simulink model "IonSatSimulationD"  (R2020b)
settings: Solver=ode3  StartTime=0.0  StopTime=t_sim  FixedStep=TimeStep  MaxStep=30  MinStep=.1  RelTol=1e-3
model workspace (MAT data in the model file):
  repartition_matrix : Simulink.Parameter (value not decoded)
  wheel_number : Simulink.Parameter (value not decoded)
values from neighbouring files (symbols this model uses):
  MODE = 4    [Full_model_PID_MEKF_Scenario1_Monte_Carlo.m]    (also in Full_model_PID_MEKF_Scenario3_Monte_Carlo.m = MODE_SEQUENCE(1); Full_model_PID_UKF_Scenario1_Monte_Carlo.m; Full_model_PID_UKF_Scenario2_Monte_Carlo.m = 2; Full_model_PID_UKF_Scenario3_Monte_Carlo.m = MODE_SEQUENCE(1))
  Use_IGRF = 1    [Full_model_PID_MEKF_Scenario1_Monte_Carlo.m]    (also in Full_model_PID_MEKF_Scenario3_Monte_Carlo.m; Full_model_PID_UKF_Scenario1_Monte_Carlo.m; Full_model_PID_UKF_Scenario2_Monte_Carlo.m; Full_model_PID_UKF_Scenario3_Monte_Carlo.m)
  Use_IGRF_KF = 1    [Full_model_PID_MEKF_Scenario1_Monte_Carlo.m]    (also in Full_model_PID_MEKF_Scenario3_Monte_Carlo.m; Full_model_PID_UKF_Scenario1_Monte_Carlo.m; Full_model_PID_UKF_Scenario2_Monte_Carlo.m; Full_model_PID_UKF_Scenario3_Monte_Carlo.m)
undefined symbols (not defined in the file or in its folder): att, date, deg, DiscIntNeverNeededParam, IonSataero, km, m, orbit, rad, s, sat
libraries: aerolibutil x30, vrlib x19, aerolibconvert2 x13, dspmathops x13, sharedtransform x12, simulink x10, sharedutil x5, DipoleModel x3, aerolibobsolete x3, simulink_extras x2, aerolibcelestial x2, dspstat3 x1
(part 3 of 3)

== system IonSatSimulationD/Sensors/Sun Sensor (Sun sensor) ==
  note: Two sensors because the top-camera has a 3-sigma=0.2° wheread the coarse sun sensors have sigma = 10°
  note: Valeur constructeur : 3-sigma = 0.2°
      | Donc sigma = 0.066° = 0.001164 rad
  note: Test d'eclipse
  note: Tests if the camera is seeing the sun
  Sat-Sun_ECI : Inport
  U : Inport  Port=2
  AND1 : Logic  IconShape=distinctive  AllPortsSameDT=off  OutDataTypeStr=boolean
  Bus Selector : BusSelector  OutputSignals=Q_ECI,XYZ_ECI
  Constant3 : Constant  Value=true
  Constant4 : Constant  Value=false
  Demux : Demux  Outputs=3
  Eclipse Test 0: in eclipse 1: illumination : MATLABFcn  MATLABFcn=eclipse_check
  Manual Switch : ManualSwitch
  Mux : Mux  Inputs=2
  Quaternion Rotation : aerolibutil/Quaternion Rotation
  Quaternion Rotation1 : aerolibutil/Quaternion Rotation
  Random Number : RandomNumber  Mean=[0 0 0]  Variance=sat.sensors.sun_sigma*sat.sensors.sun_sigma  Seed=[0 5 355]  SampleTime=1  VectorParams1D=off
  Rotation Angles to Quaternions : sharedtransform/Rotation Angles to Quaternions  rotationOrder=ZYX  aMode=aMode
      settings: SourceProductBaseCode=AE,PW,MT,UV,VE,VP
  Switch : Switch  Criteria=u2 > Threshold
  Terminator : Terminator
  Terminator1 : Terminator
  switch here to never have an eclipse : Constant
  Sat-Sun_precise_body_meas : Outport  VectorParamsAs1DForOutWhenUnconnected=off
  Sensor active (bool) : Outport  Port=2  VectorParamsAs1DForOutWhenUnconnected=off
  wires:
  Rotation Angles to Quaternions/1 -> Quaternion Rotation/1
  Quaternion Rotation/1 -> Sat-Sun_precise_body_meas/1
  U/1 -> Bus Selector/1
  Bus Selector/1 -> Quaternion Rotation1/1  "<Q_ECI>"
  Quaternion Rotation1/1 -> Demux/1, Quaternion Rotation/2  "Sat_Sun_body"
  Demux/3 -> Switch/2
  Constant3/1 -> Switch/1
  Demux/2 -> Terminator/1
  Demux/1 -> Terminator1/1
  Random Number/1 -> Rotation Angles to Quaternions/1
  Constant4/1 -> Switch/3
  Mux/1 -> Eclipse Test 0: in eclipse 1: illumination/1
  AND1/1 -> Manual Switch/1
  Bus Selector/2 -> Mux/1  "<XYZ_ECI>"
  Eclipse Test 0: in eclipse 1: illumination/1 -> AND1/2
  Switch/1 -> AND1/1
  Sat-Sun_ECI/1 -> Mux/2, Quaternion Rotation1/2
  switch here to never have an eclipse/1 -> Manual Switch/2
  Manual Switch/1 -> Sensor active (bool)/1

== system IonSatSimulationD/Attitude Controller/B-dot choice1/Switch Case Action Subsystem3 ==
  In1 : Inport
  Action Port : ActionPort  ActionPortLabel=if(u1 > 0)
  Out1 : Outport  VectorParamsAs1DForOutWhenUnconnected=off
  wires:
  In1/1 -> Out1/1

== system IonSatSimulationD/Attitude Controller/B-dot choice1/Switch Case Action Subsystem4 ==
  In1 : Inport
  Action Port : ActionPort  ActionPortLabel=else
  Out1 : Outport  VectorParamsAs1DForOutWhenUnconnected=off
  wires:
  In1/1 -> Out1/1

== system IonSatSimulationD/Attitude Controller/B-dot choice2/Switch Case Action Subsystem3 ==
  In1 : Inport
  Action Port : ActionPort  ActionPortLabel=if(u1 > 0)
  Out1 : Outport  VectorParamsAs1DForOutWhenUnconnected=off
  wires:
  In1/1 -> Out1/1

== system IonSatSimulationD/Attitude Controller/B-dot choice2/Switch Case Action Subsystem4 ==
  In1 : Inport
  Action Port : ActionPort  ActionPortLabel=else
  Out1 : Outport  VectorParamsAs1DForOutWhenUnconnected=off
  wires:
  In1/1 -> Out1/1

== system IonSatSimulationD/Attitude Controller/PID (nominal command)/Command Magnetic moments computation ==
  note: Moment magnétique de commande M :
      |
      | $M_c = \frac{1}{B²}\vec{B} \wedge\vec{T_P}$
      |
      | Avec Tp couple projeté dans le plan orthogonal à B
      | $T_P=\vec{T}-\frac{1}{B²}(\vec{T}\cdot\vec{B})\vec{B}$
  Command (vect) : Inport  OutDataTypeStr=double
  B_IGRF_body (vect) : Inport  Port=2  OutDataTypeStr=double
  h1 (vect) : Inport  Port=3
  h2 (vect) : Inport  Port=4
  h3 (vect) : Inport  Port=5
  Cross Product : vrlib/Utilities/Cross Product
  Dot Product : DotProduct  InputSameDT=on  OutDataTypeStr=Inherit: Inherit via internal rule
  Global magnetic moment computation : Subsystem
  Mux : Mux  Inputs=3
  Product1 : Product  Inputs=*/
  Reshape : Reshape  OutputDimensionality=Column vector (2-D)
  Reshape1 : Reshape  OutputDimensionality=Column vector (2-D)
  Mag vector command : Outport  VectorParamsAs1DForOutWhenUnconnected=off
  wires:
  B_IGRF_body (vect)/1 -> Reshape1/1  "B_Body"
  Command (vect)/1 -> Reshape/1  "T_Body"
  h1 (vect)/1 -> Global magnetic moment computation/2(In2)
  h2 (vect)/1 -> Global magnetic moment computation/3(In3)
  h3 (vect)/1 -> Global magnetic moment computation/4(In4)
  Global magnetic moment computation/2(magnetic moment 2 (scalar)) -> Mux/2  "magnetic moment 2"
  Global magnetic moment computation/3(magnetic moment 3 (scalar)) -> Mux/3  "magnetic moment 3"
  Global magnetic moment computation/1(magnetic moment 1 (scalar)) -> Mux/1  "magnetic moment 1"
  Mux/1 -> Mag vector command/1
  Reshape1/1 -> Cross Product/2, Dot Product/2, Dot Product/1
  Cross Product/1 -> Product1/1
  Product1/1 -> Global magnetic moment computation/1(In1)  "Mc"
  Dot Product/1 -> Product1/2  "B^2"
  Reshape/1 -> Cross Product/1  "Tp"

== system IonSatSimulationD/Attitude Controller/PID (nominal command)/Extract Vect ==
  Qr : Inport
  Demux : Demux
  Mux1 : Mux  Inputs=3
  Product : Product
  Reshape : Reshape  OutputDimensionality=Column vector (2-D)
  Sign : Signum
  Qvect : Outport  VectorParamsAs1DForOutWhenUnconnected=off
  wires:
  Demux/2 -> Mux1/1
  Demux/4 -> Mux1/3
  Demux/3 -> Mux1/2
  Demux/1 -> Sign/1
  Qr/1 -> Demux/1
  Mux1/1 -> Product/2
  Product/1 -> Reshape/1
  Sign/1 -> Product/1
  Reshape/1 -> Qvect/1

== system IonSatSimulationD/Attitude Controller/PID (nominal command)/If Action Subsystem ==
  In1 : Inport
  Action Port : ActionPort  ActionPortLabel=else
  Out1 : Outport  VectorParamsAs1DForOutWhenUnconnected=off
  wires:
  In1/1 -> Out1/1

== system IonSatSimulationD/Attitude Controller/PID (nominal command)/If Action Subsystem1 ==
  In1 : Inport
  Action Port : ActionPort  ActionPortLabel=if(u1 > 0)
  Out1 : Outport  VectorParamsAs1DForOutWhenUnconnected=off
  wires:
  In1/1 -> Out1/1

== system IonSatSimulationD/Attitude Controller/PID (nominal command)/If Action Subsystem2 ==
  In1 : Inport
  Action Port : ActionPort  ActionPortLabel=if(u1 > 0.0068)
  Out1 : Outport  VectorParamsAs1DForOutWhenUnconnected=off
  wires:
  In1/1 -> Out1/1

== system IonSatSimulationD/Attitude Controller/PID (nominal command)/If Action Subsystem3 ==
  In1 : Inport
  Action Port : ActionPort  ActionPortLabel=else
  Out1 : Outport  VectorParamsAs1DForOutWhenUnconnected=off
  wires:
  In1/1 -> Out1/1

== system IonSatSimulationD/Attitude Controller/PID (nominal command)/RW1 ==
  note: Entrées:
      | - Moment de commande (déjà projeté sur l'axe de la roue...)
      | Sorties:
      | - Omega de commande à appliquer
  Mc (scalar) : Inport
  Discrete-Time Integrator : DiscreteIntegrator  IntegratorMethod=Integration: Trapezoidal  SampleTime=-1  ICPrevOutput=DiscIntNeverNeededParam  ICPrevScaledInput=DiscIntNeverNeededParam
  Divide : Product  Inputs=*/
  Saturation_speed : Saturate  UpperLimit=sat.wheel.max_speed  LowerLimit=- sat.wheel.max_speed
  Torque_sat : Saturate  UpperLimit=sat.wheel.max_torque  LowerLimit=- sat.wheel.max_torque
  Wheel Inertia : Constant  Value=sat.wheel.max_sigma/sat.wheel.max_speed
  Omega_C (scalar) : Outport
  wires:
  Wheel Inertia/1 -> Divide/2
  Divide/1 -> Discrete-Time Integrator/1  "dw/dt"
  Discrete-Time Integrator/1 -> Saturation_speed/1
  Torque_sat/1 -> Divide/1  "Torque (scal)"
  Saturation_speed/1 -> Omega_C (scalar)/1
  Mc (scalar)/1 -> Torque_sat/1

== system IonSatSimulationD/Attitude Controller/PID (nominal command)/RW2 ==
  note: Entrées:
      | - Moment de commande (déjà projeté sur l'axe de la roue...)
      | Sorties:
      | - Omega de commande à appliquer
  Mc (scalar) : Inport
  Discrete-Time Integrator : DiscreteIntegrator  IntegratorMethod=Integration: Trapezoidal  SampleTime=-1  ICPrevOutput=DiscIntNeverNeededParam  ICPrevScaledInput=DiscIntNeverNeededParam
  Divide : Product  Inputs=*/
  Saturation_speed : Saturate  UpperLimit=sat.wheel.max_speed  LowerLimit=- sat.wheel.max_speed
  Torque_sat : Saturate  UpperLimit=sat.wheel.max_torque  LowerLimit=- sat.wheel.max_torque
  Wheel Inertia : Constant  Value=sat.wheel.max_sigma/sat.wheel.max_speed
  Omega_C (scalar) : Outport
  wires:
  Wheel Inertia/1 -> Divide/2
  Divide/1 -> Discrete-Time Integrator/1  "dw/dt"
  Discrete-Time Integrator/1 -> Saturation_speed/1
  Torque_sat/1 -> Divide/1  "Torque (scal)"
  Saturation_speed/1 -> Omega_C (scalar)/1
  Mc (scalar)/1 -> Torque_sat/1

== system IonSatSimulationD/Attitude Controller/PID (nominal command)/RW3 ==
  note: Entrées:
      | - Moment de commande (déjà projeté sur l'axe de la roue...)
      | Sorties:
      | - Omega de commande à appliquer
  Mc (scalar) : Inport
  Discrete-Time Integrator : DiscreteIntegrator  IntegratorMethod=Integration: Trapezoidal  SampleTime=-1  ICPrevOutput=DiscIntNeverNeededParam  ICPrevScaledInput=DiscIntNeverNeededParam
  Divide : Product  Inputs=*/
  Saturation_speed : Saturate  UpperLimit=sat.wheel.max_speed  LowerLimit=- sat.wheel.max_speed
  Torque_sat : Saturate  UpperLimit=sat.wheel.max_torque  LowerLimit=- sat.wheel.max_torque
  Wheel Inertia : Constant  Value=sat.wheel.max_sigma/sat.wheel.max_speed
  Omega_C (scalar) : Outport
  wires:
  Wheel Inertia/1 -> Divide/2
  Divide/1 -> Discrete-Time Integrator/1  "dw/dt"
  Discrete-Time Integrator/1 -> Saturation_speed/1
  Torque_sat/1 -> Divide/1  "Torque (scal)"
  Saturation_speed/1 -> Omega_C (scalar)/1
  Mc (scalar)/1 -> Torque_sat/1

== system IonSatSimulationD/Attitude Controller/PID (nominal command)/RW4  ==
  note: Entrées:
      | - Moment de commande (déjà projeté sur l'axe de la roue...)
      | Sorties:
      | - Omega de commande à appliquer
  Mc (scalar) : Inport
  Discrete-Time Integrator : DiscreteIntegrator  IntegratorMethod=Integration: Trapezoidal  SampleTime=-1  ICPrevOutput=DiscIntNeverNeededParam  ICPrevScaledInput=DiscIntNeverNeededParam
  Divide : Product  Inputs=*/
  Saturation_speed : Saturate  UpperLimit=sat.wheel.max_speed  LowerLimit=- sat.wheel.max_speed
  Torque_sat : Saturate  UpperLimit=sat.wheel.max_torque  LowerLimit=- sat.wheel.max_torque
  Wheel Inertia : Constant  Value=sat.wheel.max_sigma/sat.wheel.max_speed
  Omega_C (scalar) : Outport
  wires:
  Wheel Inertia/1 -> Divide/2
  Divide/1 -> Discrete-Time Integrator/1  "dw/dt"
  Discrete-Time Integrator/1 -> Saturation_speed/1
  Torque_sat/1 -> Divide/1  "Torque (scal)"
  Saturation_speed/1 -> Omega_C (scalar)/1
  Mc (scalar)/1 -> Torque_sat/1

== system IonSatSimulationD/Disturbance Torques/Aerodynamic Model/Calculate - Az & El Angle ==
  attitude : Inport
  Wind unit ECI : Inport  Port=2
  Atan2 : Trigonometry  Operator=atan2
  Constant1 : Constant  Value=2*pi
  Demux : Demux  Outputs=3
  Rotation : Product  Multiplication=Matrix(*)  RndMeth=Zero
  Sum : Sum  Inputs=|++
  Switch : Switch
  Trigonometric Function2 : Trigonometry  Operator=asin
  El : Outport
  Az : Outport  Port=2
  wires:
  attitude/1 -> Rotation/1  "ECI to BRF"
  Wind unit ECI/1 -> Rotation/2
  Rotation/1 -> Demux/1  "wind BRF"
  Demux/3 -> Trigonometric Function2/1
  Trigonometric Function2/1 -> El/1  "Elevation"
  Demux/1 -> Atan2/2
  Demux/2 -> Atan2/1
  Atan2/1 -> Switch/1, Switch/2, Sum/2
  Switch/1 -> Az/1
  Constant1/1 -> Sum/1
  Sum/1 -> Switch/3

== system IonSatSimulationD/Disturbance Torques/Aerodynamic Model/Get Density ==
  note: Altitude (distance to center of earth)
  <XYZ_ECI> : Inport
  DOY : Inport  Port=2
  "DCM_i2e " : Inport  Port=3
  Demux1 : Demux  Outputs=3
  Dot Product - magnitude squared : DotProduct  InputSameDT=on  OutDataTypeStr=Inherit: Inherit via internal rule
  ECI To LLA : MATLAB Function  TreatAsAtomicUnit=on
  Lookup - Air density : Lookup  InputValues=IonSataero.alt_range*1000 + 6378100  Table=IonSataero.av_density_vs_alt
  MATLAB Function2 : MATLAB Function  TreatAsAtomicUnit=on
  Mux2 : Mux  Inputs=3
  NRLMSISE-00 Atmosphere Model : aerolibatmos2/NRLMSISE-00 Atmosphere Model  units=Metric (MKS)  lst_input=off  flux_ap_input=off  flags_input=Internal  flags=ones(1,23)  oxygen_in=on  action=Warning
      settings: SourceProductBaseCode=AE
  Product : Product  Multiplication=Matrix(*)
  Reshape : Reshape  OutputDimensionality=Row vector (2-D)
  Scope : Scope  NumInputPorts=2
  Terminator : Terminator
  sqrt : Math  Operator=sqrt  SignedPower=on  SaturateOnIntegerOverflow=on
  Density Lookup table : Outport
  Density NRLMSISE : Outport  Port=2
  wires:
  Dot Product - magnitude squared/1 -> sqrt/1
  Lookup - Air density/1 -> Scope/1, Density Lookup table/1  "Density Lookup"
  sqrt/1 -> Lookup - Air density/1
  DOY/1 -> Demux1/1
  Demux1/1 -> NRLMSISE-00 Atmosphere Model/2
  Demux1/2 -> NRLMSISE-00 Atmosphere Model/3
  NRLMSISE-00 Atmosphere Model/2 -> MATLAB Function2/1(u)
  Demux1/3 -> NRLMSISE-00 Atmosphere Model/4
  Mux2/1 -> NRLMSISE-00 Atmosphere Model/1
  NRLMSISE-00 Atmosphere Model/1 -> Terminator/1
  MATLAB Function2/1(y) -> Scope/2, Density NRLMSISE/1  "Density NRLMSISE"
  Reshape/1 -> Product/1
  "DCM_i2e "/1 -> Product/2  "DCM_i2e"
  <XYZ_ECI>/1 -> Reshape/1, Dot Product - magnitude squared/1, Dot Product - magnitude squared/2
  Product/1 -> ECI To LLA/1(X_ECEF)
  ECI To LLA/2(lat) -> Mux2/1
  ECI To LLA/3(long) -> Mux2/2
  ECI To LLA/1(h) -> Mux2/3

== system IonSatSimulationD/IGRF Computation block/Obtain B_ECI/Dipole Subsystem ==
  In1 : Inport
  Action Port : ActionPort  ActionPortLabel=else
  Bus Selector1 : BusSelector  OutputSignals=h,lat,long,DCM_i2e
  Dipole Model : DipoleModel/Dipole Model  SystemSampleTime=-1  VariantActivationTime=update diagram  Latency=0  AutoFrameSizeCalculation=off
  Out1 : Outport  VectorParamsAs1DForOutWhenUnconnected=off
  wires:
  In1/1 -> Bus Selector1/1
  Bus Selector1/3 -> Dipole Model/3  "<long>"
  Dipole Model/1 -> Out1/1
  Bus Selector1/1 -> Dipole Model/1  "<h>"
  Bus Selector1/2 -> Dipole Model/2  "<lat>"
  Bus Selector1/4 -> Dipole Model/4  "<DCM_i2e>"

== system IonSatSimulationD/IGRF Computation block/Obtain B_ECI/IGRF Subsystem ==
  In1 : Inport
  Action Port : ActionPort  ActionPortLabel=if(u1 > 0)
  Bus Selector : BusSelector  OutputSignals=DCM_i2e,h,lat,long,signal4
  International Geomagnetic Reference Field 12 : aerolibobsolete/International Geomagnetic Reference Field 12  units=Metric (MKS)  time_in=on  month=January  day=1  year=2020  action=None  sv_out=on
      settings: SourceProductBaseCode=AE
  Mux : Mux  Inputs=3
  NED to ECEF : MATLABFcn  MATLABFcn=NED2ecef  OutputDimensions=[3;1]  Output1D=off
  Permute Dimensions : PermuteDimensions
  Product : Product  Multiplication=Matrix(*)
  T to nT : Gain  Gain=1E-9
  Terminator{1..9} (9 alike) : Terminator
  Out1 : Outport  VectorParamsAs1DForOutWhenUnconnected=off
  wires:
  In1/1 -> Bus Selector/1
  Bus Selector/2 -> International Geomagnetic Reference Field 12/1  "<h>"
  T to nT/1 -> Out1/1
  Bus Selector/5 -> International Geomagnetic Reference Field 12/4  "<signal4>"
  Bus Selector/4 -> Mux/3, International Geomagnetic Reference Field 12/3  "<long>"
  Bus Selector/3 -> Mux/2, International Geomagnetic Reference Field 12/2  "<lat>"
  International Geomagnetic Reference Field 12/2 -> Terminator1/1
  International Geomagnetic Reference Field 12/10 -> Terminator9/1
  International Geomagnetic Reference Field 12/4 -> Terminator3/1
  International Geomagnetic Reference Field 12/5 -> Terminator4/1
  International Geomagnetic Reference Field 12/3 -> Terminator2/1
  International Geomagnetic Reference Field 12/1 -> Mux/1
  International Geomagnetic Reference Field 12/6 -> Terminator5/1
  International Geomagnetic Reference Field 12/8 -> Terminator7/1
  International Geomagnetic Reference Field 12/7 -> Terminator6/1
  International Geomagnetic Reference Field 12/9 -> Terminator8/1
  Bus Selector/1 -> Permute Dimensions/1  "<DCM_i2e>"
  Permute Dimensions/1 -> Product/1
  Product/1 -> T to nT/1
  Mux/1 -> NED to ECEF/1
  NED to ECEF/1 -> Product/2

== system IonSatSimulationD/Kalman Filter/IGRF Computation block orig/Obtain B_ECI ==
  In1 : Inport
  Dipole Subsystem : Subsystem  TreatAsAtomicUnit=on
  IGRF Subsystem : Subsystem  TreatAsAtomicUnit=on
  If : If
  Merge : Merge
  Use_IGRF : Constant  Value=Use_IGRF_KF
  Out1 : Outport  VectorParamsAs1DForOutWhenUnconnected=off
  wires:
  If/1 -> IGRF Subsystem/Action
  In1/1 -> Dipole Subsystem/1(In1), IGRF Subsystem/1(In1)
  IGRF Subsystem/1(Out1) -> Merge/1
  Use_IGRF/1 -> If/1
  Merge/1 -> Out1/1
  Dipole Subsystem/1(Out1) -> Merge/2
  If/2 -> Dipole Subsystem/Action

== system IonSatSimulationD/Kalman Filter/IGRF Computation block1/Obtain B_ECI ==
  In1 : Inport
  Dipole Subsystem : Subsystem  TreatAsAtomicUnit=on
  IGRF Subsystem : Subsystem  TreatAsAtomicUnit=on
  If : If
  Merge : Merge
  Use_IGRF : Constant  Value=Use_IGRF
  Out1 : Outport  VectorParamsAs1DForOutWhenUnconnected=off
  wires:
  If/1 -> IGRF Subsystem/Action
  In1/1 -> Dipole Subsystem/1(In1), IGRF Subsystem/1(In1)
  IGRF Subsystem/1(Out1) -> Merge/1
  Use_IGRF/1 -> If/1
  Merge/1 -> Out1/1
  Dipole Subsystem/1(Out1) -> Merge/2
  If/2 -> Dipole Subsystem/Action

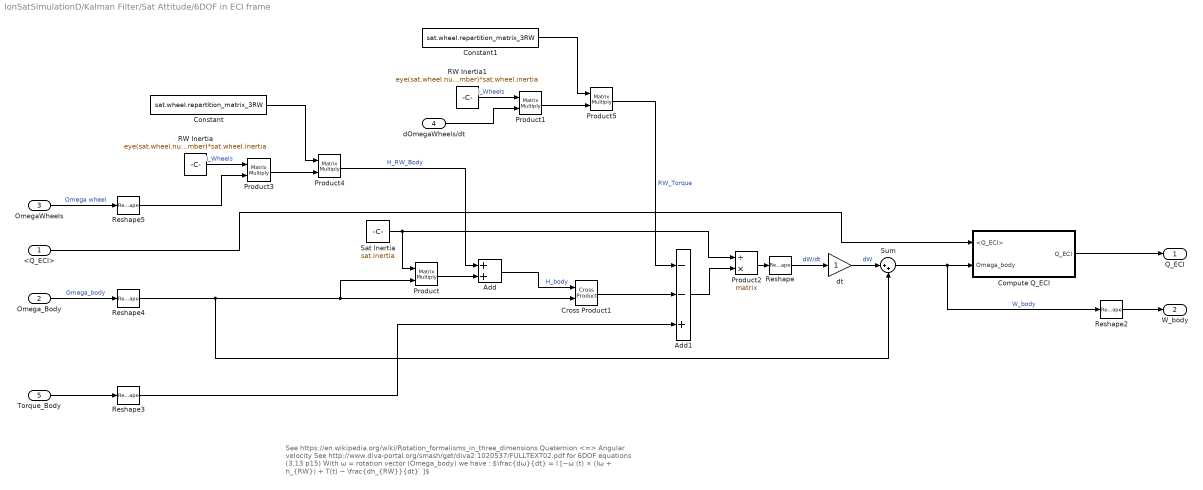
== system IonSatSimulationD/Kalman Filter/Sat Attitude/6DOF in ECI frame ==
  note: See https://en.wikipedia.org/wiki/Rotation_formalisms_in_three_dimensions Quaternion <=> Angular velocity
      |
      | See http://www.diva-portal.org/smash/get/diva2:1020537/FULLTEXT02.pdf for 6DOF equations (3.13 p15)
      |
      | With ω = rotation vector (Omega_body) we have :
      |
      | $\frac{dω}{dt} = I [−ω (t) × (Iω + h_{RW}) + T(t) − \frac{dh_{RW}}{dt} ̇ ]$
  <Q_ECI> : Inport
  "Omega_Body " : Inport  Port=2
  OmegaWheels : Inport  Port=3
  dOmegaWheels/dt : Inport  Port=4
  Torque_Body : Inport  Port=5
  Add : Sum
  Add1 : Sum  Inputs=--+
  Compute Q_ECI : Subsystem
  Constant : Constant  Value=sat.wheel.repartition_matrix_3RW
  Constant1 : Constant  Value=sat.wheel.repartition_matrix_3RW
  Cross Product1 : vrlib/Utilities/Cross Product
  Product{,1,3..5} (5 alike) : Product  Multiplication=Matrix(*)
  Product2 : Product  Inputs=/*  Multiplication=Matrix(*)
  RW Inertia : Constant  Value=eye(sat.wheel.number)*sat.wheel.inertia
  RW Inertia1 : Constant  Value=eye(sat.wheel.number)*sat.wheel.inertia
  Reshape : Reshape
  Reshape2 : Reshape
  Reshape3 : Reshape  OutputDimensionality=Column vector (2-D)
  Reshape4 : Reshape  OutputDimensionality=Column vector (2-D)
  Reshape5 : Reshape  OutputDimensionality=Column vector (2-D)
  Sat Inertia : Constant  Value=sat.inertia
  Sum : Sum  Inputs=|++
  dt : Gain
  Q_ECI : Outport  VectorParamsAs1DForOutWhenUnconnected=off
  W_body : Outport  Port=2  VectorParamsAs1DForOutWhenUnconnected=off
  wires:
  Product2/1 -> Reshape/1
  Product3/1 -> Product4/2
  Sat Inertia/1 -> Product/1, Product2/1
  Add/1 -> Cross Product1/1  "H_body"
  Add1/1 -> Product2/2
  Cross Product1/1 -> Add1/2
  "Omega_Body "/1 -> Reshape4/1  "Omega_body"
  Product/1 -> Add/2
  RW Inertia/1 -> Product3/1  "I_Wheels"
  Torque_Body/1 -> Reshape3/1
  Product5/1 -> Add1/1  "RW_Torque"
  OmegaWheels/1 -> Reshape5/1  "Omega wheel"
  Constant/1 -> Product4/1
  Product4/1 -> Add/1  "H_RW_Body"
  Reshape3/1 -> Add1/3
  Reshape/1 -> dt/1  "dW/dt"
  Sum/1 -> Compute Q_ECI/2(Omega_body), Reshape2/1  "W_body"
  Compute Q_ECI/1(Q_ECI) -> Q_ECI/1
  Reshape2/1 -> W_body/1
  Reshape4/1 -> Sum/2, Cross Product1/2, Product/2
  Reshape5/1 -> Product3/2
  <Q_ECI>/1 -> Compute Q_ECI/1(<Q_ECI>)
  dt/1 -> Sum/1  "dW"
  dOmegaWheels/dt/1 -> Product1/2
  Constant1/1 -> Product5/1
  Product1/1 -> Product5/2
  RW Inertia1/1 -> Product1/1  "I_Wheels"

== system IonSatSimulationD/Kalman Filter/Sat Attitude/Magnetorquer physics ==
  note: On pourrait aussi changer les blocs
      | magnétocoupleurs pour sortir les intensités
  Mag vector command : Inport
  B_IGRF_body (vecteur) : Inport  Port=2
  Add1 : Sum  Inputs=+++
  Cross Product : vrlib/Utilities/Cross Product
  Demux : Demux  Outputs=3
  Magnétocoupleur 1 : Subsystem
  Magnétocoupleur 2 : Subsystem
  Magnétocoupleur 3 : Subsystem
  Couple (vect) : Outport  VectorParamsAs1DForOutWhenUnconnected=off
  wires:
  Add1/1 -> Cross Product/1  "M_real"
  Demux/1 -> Magnétocoupleur 1/1(m_in (scalar))
  Demux/2 -> Magnétocoupleur 2/1(m_in (scalar))
  Demux/3 -> Magnétocoupleur 3/1(m_in (scalar))
  Mag vector command/1 -> Demux/1
  Magnétocoupleur 2/1(m_out (vect)) -> Add1/2
  Magnétocoupleur 1/1(m_out (vect)) -> Add1/1
  Magnétocoupleur 3/1(m_out (vect)) -> Add1/3
  Cross Product/1 -> Couple (vect)/1  "T_body"
  B_IGRF_body (vecteur)/1 -> Cross Product/2

== system IonSatSimulationD/Kalman Filter/Sat Attitude1/Compute Q_ECI ==
  note: https://arxiv.org/pdf/0811.2889.pdf
      | $ω = 2q^*\frac{dq}{dt}$ (13)
      |
      | $\frac{dq}{dt} = \frac{1}{2} q * ω$ (14)
  <Q_ECI> : Inport
  Omega_body : Inport  Port=2
  Gain : Gain  Gain=1/2
  Ground : Ground
  Mux : Mux  Inputs=2
  Quaternion Multiplication : aerolibutil/Quaternion Multiplication
  Quaternion Normalize : sharedutil/Quaternion Normalize  aMode=aMode
      settings: SourceProductBaseCode=AE,PW,MT,UV,VE,VP
  Sum : Sum  Inputs=|++
  dt : Gain
  Q_ECI : Outport  VectorParamsAs1DForOutWhenUnconnected=off
  wires:
  Quaternion Multiplication/1 -> Gain/1
  Omega_body/1 -> Mux/2
  Ground/1 -> Mux/1
  Mux/1 -> Quaternion Multiplication/2
  Quaternion Normalize/1 -> Q_ECI/1  "Q_ECI"
  Sum/1 -> Quaternion Normalize/1
  <Q_ECI>/1 -> Quaternion Multiplication/1, Sum/1
  Gain/1 -> dt/1  "dQ"
  dt/1 -> Sum/2

== system IonSatSimulationD/Physical Model/6DOF in ECI frame/Compute Omega ==
  note: https://arxiv.org/pdf/0811.2889.pdf
      | $ω = 2q^*\frac{dq}{dt}$ (13)
  <Q_ECI> : Inport
  Demux : Demux  Outputs=2
  Derivative : Derivative
  Gain : Gain  Gain=2
  Quaternion Conjugate : aerolibutil/Quaternion Conjugate
      settings: SourceProductBaseCode=AE
  Quaternion Multiplication : aerolibutil/Quaternion Multiplication
  Reshape : Reshape  OutputDimensionality=Column vector (2-D)
  Terminator : Terminator
  Omega_body : Outport  PortDimensions=[3 1]  VectorParamsAs1DForOutWhenUnconnected=off
  wires:
  Quaternion Multiplication/1 -> Demux/1
  <Q_ECI>/1 -> Derivative/1, Quaternion Conjugate/1
  Demux/1 -> Terminator/1
  Demux/2 -> Reshape/1
  Reshape/1 -> Gain/1
  Gain/1 -> Omega_body/1
  Quaternion Conjugate/1 -> Quaternion Multiplication/1
  Derivative/1 -> Quaternion Multiplication/2

== system IonSatSimulationD/Physical Model/6DOF in ECI frame/Compute Q_ECI ==
  note: https://arxiv.org/pdf/0811.2889.pdf
      | $ω = 2q^*\frac{dq}{dt}$ (13)
      |
      | $\frac{dq}{dt} = \frac{1}{2} q * ω$ (14)
  <Q_ECI> : Inport
  Omega_body : Inport  Port=2
  Gain : Gain  Gain=1/2
  Ground : Ground
  Integrator_quat : Integrator  InitialCondition=[1 0 0 0]
  Mux : Mux  Inputs=2
  Quaternion Multiplication : aerolibutil/Quaternion Multiplication
  Quaternion Normalize : sharedutil/Quaternion Normalize  aMode=aMode
      settings: SourceProductBaseCode=AE,PW,MT,UV,VE,VP
  Q_ECI : Outport  VectorParamsAs1DForOutWhenUnconnected=off
  wires:
  Quaternion Multiplication/1 -> Gain/1
  Omega_body/1 -> Mux/2
  Ground/1 -> Mux/1
  Mux/1 -> Quaternion Multiplication/2
  <Q_ECI>/1 -> Quaternion Multiplication/1
  Integrator_quat/1 -> Quaternion Normalize/1
  Gain/1 -> Integrator_quat/1
  Quaternion Normalize/1 -> Q_ECI/1  "Q_ECI"

== system IonSatSimulationD/Physical Model/Magnetorquer physics/Magnétocoupleur 1 ==
  note: les grounds représentant les limites en
      |  moment magnétique du magnétocoupleur (lié à l'intensité)
      | A définir
  m_in (scalar) : Inport
  Constant1 : Constant  Value=sat.mag_t.max_mm1
  Constant2 : Constant  Value=- sat.mag_t.max_mm1
  Constant6 : Constant  Value=sat.mag_t.axe1
  Product : Product
  Saturation Dynamic : simulink/Discontinuities/Saturation Dynamic  OutMin=[]  OutMax=[]  OutDataTypeStr=Inherit: Same as second input  OutDataType=fixdt(1, 16)  OutScaling=2^-10  DoSatur=off
  m_out (vect) : Outport  VectorParamsAs1DForOutWhenUnconnected=off
  wires:
  m_in (scalar)/1 -> Saturation Dynamic/2
  Constant2/1 -> Saturation Dynamic/3
  Constant1/1 -> Saturation Dynamic/1
  Saturation Dynamic/1 -> Product/1
  Product/1 -> m_out (vect)/1
  Constant6/1 -> Product/2

== system IonSatSimulationD/Physical Model/Magnetorquer physics/Magnétocoupleur 2 ==
  note: les grounds représentant les limites en
      |  moment magnétique du magnétocoupleur (lié à l'intensité)
      | A définir
  m_in (scalar) : Inport
  Constant : Constant  Value=- sat.mag_t.max_mm2
  Constant1 : Constant  Value=sat.mag_t.max_mm2
  Constant6 : Constant  Value=sat.mag_t.axe2
  Product : Product
  Saturation Dynamic : simulink/Discontinuities/Saturation Dynamic  OutMin=[]  OutMax=[]  OutDataTypeStr=Inherit: Same as second input  OutDataType=fixdt(1, 16)  OutScaling=2^-10  DoSatur=off
  m_out (vect) : Outport  VectorParamsAs1DForOutWhenUnconnected=off
  wires:
  m_in (scalar)/1 -> Saturation Dynamic/2
  Constant/1 -> Saturation Dynamic/3
  Constant1/1 -> Saturation Dynamic/1
  Product/1 -> m_out (vect)/1
  Constant6/1 -> Product/2
  Saturation Dynamic/1 -> Product/1

== system IonSatSimulationD/Physical Model/Magnetorquer physics/Magnétocoupleur 3 ==
  note: les grounds représentant les limites en
      |  moment magnétique du magnétocoupleur (lié à l'intensité)
      | A définir
  m_in (scalar) : Inport
  Constant1 : Constant  Value=sat.mag_t.max_mm3
  Constant2 : Constant  Value=- sat.mag_t.max_mm3
  Constant6 : Constant  Value=sat.mag_t.axe3
  Product : Product
  Saturation Dynamic : simulink/Discontinuities/Saturation Dynamic  OutMin=[]  OutMax=[]  OutDataTypeStr=Inherit: Same as second input  OutDataType=fixdt(1, 16)  OutScaling=2^-10  DoSatur=off
  m_out (vect) : Outport  VectorParamsAs1DForOutWhenUnconnected=off
  wires:
  m_in (scalar)/1 -> Saturation Dynamic/2
  Constant2/1 -> Saturation Dynamic/3
  Constant1/1 -> Saturation Dynamic/1
  Product/1 -> m_out (vect)/1
  Constant6/1 -> Product/2
  Saturation Dynamic/1 -> Product/1

== system IonSatSimulationD/Physical Model/Thruster/If Action Subsystem ==
  In1 : Inport
  Action Port : ActionPort  ActionPortLabel=if(u1)
  Out1 : Outport
  wires:
  In1/1 -> Out1/1

== system IonSatSimulationD/Physical Model/Thruster/If Action Subsystem1 ==
  In1 : Inport
  Action Port : ActionPort  ActionPortLabel=else
  Out1 : Outport
  wires:
  In1/1 -> Out1/1

== system IonSatSimulationD/Attitude Controller/PID (nominal command)/Command Magnetic moments computation/Global magnetic moment computation ==
  In1 : Inport  OutDataTypeStr=double
  In2 : Inport  Port=2
  In3 : Inport  Port=3
  In4 : Inport  Port=4
  Dot Product : DotProduct  InputSameDT=on  OutDataTypeStr=Inherit: Inherit via internal rule
  Dot Product1 : DotProduct  InputSameDT=on  OutDataTypeStr=Inherit: Inherit via internal rule
  Dot Product2 : DotProduct  InputSameDT=on  OutDataTypeStr=Inherit: Inherit via internal rule
  magnetic moment 1 (scalar) : Outport
  magnetic moment 2 (scalar) : Outport  Port=2
  magnetic moment 3 (scalar) : Outport  Port=3
  wires:
  In1/1 -> Dot Product2/1, Dot Product1/1, Dot Product/1
  In2/1 -> Dot Product/2
  In3/1 -> Dot Product1/2
  In4/1 -> Dot Product2/2
  Dot Product/1 -> magnetic moment 1 (scalar)/1
  Dot Product1/1 -> magnetic moment 2 (scalar)/1
  Dot Product2/1 -> magnetic moment 3 (scalar)/1

== system IonSatSimulationD/Kalman Filter/IGRF Computation block orig/Obtain B_ECI/Dipole Subsystem ==
  In1 : Inport
  Action Port : ActionPort
  Bus Selector1 : BusSelector  OutputSignals=h,lat,long,DCM_i2e
  Dipole Model : DipoleModel/Dipole Model  SystemSampleTime=-1  VariantActivationTime=update diagram  Latency=0  AutoFrameSizeCalculation=off
  Out1 : Outport  VectorParamsAs1DForOutWhenUnconnected=off
  wires:
  In1/1 -> Bus Selector1/1
  Bus Selector1/3 -> Dipole Model/3  "<long>"
  Dipole Model/1 -> Out1/1
  Bus Selector1/1 -> Dipole Model/1  "<h>"
  Bus Selector1/2 -> Dipole Model/2  "<lat>"
  Bus Selector1/4 -> Dipole Model/4  "<DCM_i2e>"

== system IonSatSimulationD/Kalman Filter/IGRF Computation block orig/Obtain B_ECI/IGRF Subsystem ==
  In1 : Inport
  Action Port : ActionPort
  Bus Selector : BusSelector  OutputSignals=DCM_i2e,h,lat,long,signal4
  International Geomagnetic Reference Field 12 : aerolibobsolete/International Geomagnetic Reference Field 12  units=Metric (MKS)  time_in=on  month=January  day=1  year=2020  action=None  sv_out=on
      settings: SourceProductBaseCode=AE
  T to nT : Gain  Gain=1E-9
  Terminator{1..9} (9 alike) : Terminator
  Out1 : Outport  VectorParamsAs1DForOutWhenUnconnected=off
  wires:
  In1/1 -> Bus Selector/1
  Bus Selector/2 -> International Geomagnetic Reference Field 12/1  "<h>"
  T to nT/1 -> Out1/1
  Bus Selector/5 -> International Geomagnetic Reference Field 12/4  "<signal4>"
  Bus Selector/4 -> International Geomagnetic Reference Field 12/3  "<long>"
  Bus Selector/3 -> International Geomagnetic Reference Field 12/2  "<lat>"
  International Geomagnetic Reference Field 12/2 -> Terminator1/1
  International Geomagnetic Reference Field 12/10 -> Terminator9/1
  International Geomagnetic Reference Field 12/4 -> Terminator3/1
  International Geomagnetic Reference Field 12/5 -> Terminator4/1
  International Geomagnetic Reference Field 12/3 -> Terminator2/1
  International Geomagnetic Reference Field 12/6 -> Terminator5/1
  International Geomagnetic Reference Field 12/8 -> Terminator7/1
  International Geomagnetic Reference Field 12/7 -> Terminator6/1
  International Geomagnetic Reference Field 12/9 -> Terminator8/1
  International Geomagnetic Reference Field 12/1 -> T to nT/1

== system IonSatSimulationD/Kalman Filter/IGRF Computation block1/Obtain B_ECI/Dipole Subsystem ==
  In1 : Inport
  Action Port : ActionPort  ActionPortLabel=else
  Bus Selector1 : BusSelector  OutputSignals=h,lat,long,DCM_i2e
  Dipole Model : DipoleModel/Dipole Model  SystemSampleTime=-1  VariantActivationTime=update diagram  Latency=0  AutoFrameSizeCalculation=off
  Out1 : Outport  VectorParamsAs1DForOutWhenUnconnected=off
  wires:
  In1/1 -> Bus Selector1/1
  Bus Selector1/3 -> Dipole Model/3  "<long>"
  Dipole Model/1 -> Out1/1
  Bus Selector1/1 -> Dipole Model/1  "<h>"
  Bus Selector1/2 -> Dipole Model/2  "<lat>"
  Bus Selector1/4 -> Dipole Model/4  "<DCM_i2e>"

== system IonSatSimulationD/Kalman Filter/IGRF Computation block1/Obtain B_ECI/IGRF Subsystem ==
  In1 : Inport
  Action Port : ActionPort  ActionPortLabel=if(u1 > 0)
  Bus Selector : BusSelector  OutputSignals=DCM_i2e,h,lat,long,signal4
  International Geomagnetic Reference Field 12 : aerolibobsolete/International Geomagnetic Reference Field 12  units=Metric (MKS)  time_in=on  month=January  day=1  year=2020  action=None  sv_out=on
      settings: SourceProductBaseCode=AE
  Mux : Mux  Inputs=3
  NED to ECEF : MATLABFcn  MATLABFcn=NED2ecef  OutputDimensions=[3;1]  Output1D=off
  Permute Dimensions : PermuteDimensions
  Product : Product  Multiplication=Matrix(*)
  T to nT : Gain  Gain=1E-9
  Terminator{1..9} (9 alike) : Terminator
  Out1 : Outport  VectorParamsAs1DForOutWhenUnconnected=off
  wires:
  In1/1 -> Bus Selector/1
  Bus Selector/2 -> International Geomagnetic Reference Field 12/1  "<h>"
  T to nT/1 -> Out1/1
  Bus Selector/5 -> International Geomagnetic Reference Field 12/4  "<signal4>"
  Bus Selector/4 -> Mux/3, International Geomagnetic Reference Field 12/3  "<long>"
  Bus Selector/3 -> Mux/2, International Geomagnetic Reference Field 12/2  "<lat>"
  International Geomagnetic Reference Field 12/2 -> Terminator1/1
  International Geomagnetic Reference Field 12/10 -> Terminator9/1
  International Geomagnetic Reference Field 12/4 -> Terminator3/1
  International Geomagnetic Reference Field 12/5 -> Terminator4/1
  International Geomagnetic Reference Field 12/3 -> Terminator2/1
  International Geomagnetic Reference Field 12/1 -> Mux/1
  International Geomagnetic Reference Field 12/6 -> Terminator5/1
  International Geomagnetic Reference Field 12/8 -> Terminator7/1
  International Geomagnetic Reference Field 12/7 -> Terminator6/1
  International Geomagnetic Reference Field 12/9 -> Terminator8/1
  Bus Selector/1 -> Permute Dimensions/1  "<DCM_i2e>"
  Permute Dimensions/1 -> Product/1
  Product/1 -> T to nT/1
  Mux/1 -> NED to ECEF/1
  NED to ECEF/1 -> Product/2

== system IonSatSimulationD/Kalman Filter/Sat Attitude/6DOF in ECI frame/Compute Q_ECI ==
  note: https://arxiv.org/pdf/0811.2889.pdf
      | $ω = 2q^*\frac{dq}{dt}$ (13)
      |
      | $\frac{dq}{dt} = \frac{1}{2} q * ω$ (14)
  <Q_ECI> : Inport
  Omega_body : Inport  Port=2
  Gain : Gain  Gain=1/2
  Ground : Ground
  Mux : Mux  Inputs=2
  Quaternion Multiplication : aerolibutil/Quaternion Multiplication
  Quaternion Normalize : sharedutil/Quaternion Normalize  aMode=aMode
      settings: SourceProductBaseCode=AE,PW,MT,UV,VE,VP
  Sum : Sum  Inputs=|++
  dt : Gain
  Q_ECI : Outport  VectorParamsAs1DForOutWhenUnconnected=off
  wires:
  Quaternion Multiplication/1 -> Gain/1
  Omega_body/1 -> Mux/2
  Ground/1 -> Mux/1
  Mux/1 -> Quaternion Multiplication/2
  Quaternion Normalize/1 -> Q_ECI/1  "Q_ECI"
  Sum/1 -> Quaternion Normalize/1
  <Q_ECI>/1 -> Quaternion Multiplication/1, Sum/1
  Gain/1 -> dt/1  "dQ"
  dt/1 -> Sum/2

== system IonSatSimulationD/Kalman Filter/Sat Attitude/Magnetorquer physics/Magnétocoupleur 1 ==
  note: les grounds représentant les limites en
      |  moment magnétique du magnétocoupleur (lié à l'intensité)
      | A définir
  m_in (scalar) : Inport
  Constant1 : Constant  Value=sat.mag_t.max_mm1
  Constant2 : Constant  Value=- sat.mag_t.max_mm1
  Constant6 : Constant  Value=sat.mag_t.axe1
  Product : Product
  Saturation Dynamic : simulink/Discontinuities/Saturation Dynamic  OutMin=[]  OutMax=[]  OutDataTypeStr=Inherit: Same as second input  OutDataType=fixdt(1, 16)  OutScaling=2^-10  DoSatur=off
  m_out (vect) : Outport  VectorParamsAs1DForOutWhenUnconnected=off
  wires:
  m_in (scalar)/1 -> Saturation Dynamic/2
  Constant2/1 -> Saturation Dynamic/3
  Constant1/1 -> Saturation Dynamic/1
  Saturation Dynamic/1 -> Product/1
  Product/1 -> m_out (vect)/1
  Constant6/1 -> Product/2

== system IonSatSimulationD/Kalman Filter/Sat Attitude/Magnetorquer physics/Magnétocoupleur 2 ==
  note: les grounds représentant les limites en
      |  moment magnétique du magnétocoupleur (lié à l'intensité)
      | A définir
  m_in (scalar) : Inport
  Constant : Constant  Value=- sat.mag_t.max_mm2
  Constant1 : Constant  Value=sat.mag_t.max_mm2
  Constant6 : Constant  Value=sat.mag_t.axe2
  Product : Product
  Saturation Dynamic : simulink/Discontinuities/Saturation Dynamic  OutMin=[]  OutMax=[]  OutDataTypeStr=Inherit: Same as second input  OutDataType=fixdt(1, 16)  OutScaling=2^-10  DoSatur=off
  m_out (vect) : Outport  VectorParamsAs1DForOutWhenUnconnected=off
  wires:
  m_in (scalar)/1 -> Saturation Dynamic/2
  Constant/1 -> Saturation Dynamic/3
  Constant1/1 -> Saturation Dynamic/1
  Product/1 -> m_out (vect)/1
  Constant6/1 -> Product/2
  Saturation Dynamic/1 -> Product/1

== system IonSatSimulationD/Kalman Filter/Sat Attitude/Magnetorquer physics/Magnétocoupleur 3 ==
  note: les grounds représentant les limites en
      |  moment magnétique du magnétocoupleur (lié à l'intensité)
      | A définir
  m_in (scalar) : Inport
  Constant1 : Constant  Value=sat.mag_t.max_mm3
  Constant2 : Constant  Value=- sat.mag_t.max_mm3
  Constant6 : Constant  Value=sat.mag_t.axe3
  Product : Product
  Saturation Dynamic : simulink/Discontinuities/Saturation Dynamic  OutMin=[]  OutMax=[]  OutDataTypeStr=Inherit: Same as second input  OutDataType=fixdt(1, 16)  OutScaling=2^-10  DoSatur=off
  m_out (vect) : Outport  VectorParamsAs1DForOutWhenUnconnected=off
  wires:
  m_in (scalar)/1 -> Saturation Dynamic/2
  Constant2/1 -> Saturation Dynamic/3
  Constant1/1 -> Saturation Dynamic/1
  Product/1 -> m_out (vect)/1
  Constant6/1 -> Product/2
  Saturation Dynamic/1 -> Product/1

== matlab function IonSatSimulationD/Time propagator/MATLAB Function ==
  data: t input; Y output; DOY output; S output
function [Y, DOY, S] = DOY(t)
Y = 2022 + fix(t/31557600);
DOY = 1+fix((t-floor(t/31557600)*31557600)/86400);
S = t - fix(t/31557600)*31557600 - (DOY-1)*86400;

== matlab function IonSatSimulationD/Kalman Filter/IGRF Computation block orig/ECI To LLA ==
  data: X_ECEF input; h output; lat output; long output
function [h, lat, long] = fcn(X_ECEF)
    h = 0;
    lat = 0;
    long = 0;
[lat, long, h] = ecef2geod(X_ECEF(1),X_ECEF(2),X_ECEF(3));

== matlab function IonSatSimulationD/Initialize Function/orb2rv ==
  data: a input; r output; e input; i input; O input; o input; nu input; v output; truLon input; argLat input; lonPer input
%----------------------- Begin Code Sequence -----------------------------%
% Purpose:                                                                %
% Convert a given set of Keplerian Orbital Elements to state vectors in   %
% in the ECI frame of reference                                           %
%                                                                         %
%-------------------------------------------------------------------------%
%                                                                         %
% Inputs:                                                                 %
%-------- 
%a                      [1 x N]                         Semimajor axis
%                                                       (km)
%
%e                      [1 x N]                         Eccentricity Magnitude
%                                                       (unitless)
%
%i                      [1 x N]                         inclination
%                                                       (radians)
%
%O                      [1 x N]                         Right Ascention of
%                                                       the ascending node
%                                                       (radians)
%
%o                      [1 x N]                         Argument of perigee
%                                                       (radians)
%
%nu                     [1 x N]                         True Anomaly
%                                                       (radians)
%
%truLon                 [1 x N]                         True Longitude
%                                                       (radians)
%
%argLat                 [1 x N]                         Argument of Latitude
%                                                       (radians)
%
%lonPer                 [1 x N]                         Longitude of Periapse
%                                                       (radians)
%
%mu                     double                          Gravitational Constant
%                                                       Defaults to Earth if
%                                                       not specified
%
% Outputs:
%---------                                                                %
%r_ECI                  [3 x N]                         Position Vector in
%                                                       ECI coordinate
%                                                       frame of reference
%
%v_ECI                  [3 x N]                         Velocity vector in
%                                                       ECI coordinate
%                                                       frame of reference
%
% References:
%-------------
%Vallado,D. Fundamentals of Astrodynamics and Applications. 2007.
%
% Function Dependencies:
%------------------
%None
%------------------------------------------------------------------       %
% Programed by Darin Koblick  03-04-2012                                  %
%------------------------------------------------------------------       %
function [r,v] = orb2rv(a,e,i,O,o,nu,truLon,argLat,lonPer)
mu = 398600.4418;
%Make all inputs consistent w/ dimensions
a = a(:); e = e(:); i = i(:); O = O(:); o = o(:); nu = nu(:);
if e<1
    p=a*(1-e*e);
else
    p=2*a;
end
ietol = 1e-8;
idx = e < ietol & mod(i,pi) < ietol;
if any(idx); o(idx) = 0; O(idx) = 0; nu(idx) = truLon(idx); end
idx = e < ietol & mod(i,pi) > ietol;
if any(idx); o(idx) = 0; nu(idx) = argLat(idx); end
idx = e > ietol & mod(i,pi) < ietol;
if any(idx); O(idx) = 0; o(idx) = lonPer(idx); end
%Find rPQW and vPQW
rPQW = cat(2,p.*cos(nu)./(1 +e.*cos(nu)),p.*sin(nu)./(1+e.*cos(nu)),zeros(size(nu)));
vPQW = cat(2,-sqrt(mu./p).*sin(nu),sqrt(mu./p).*(e+cos(nu)),zeros(size(nu)));
%Create Transformation Matrix
PQW2IJK = NaN(3,3,size(p,1));
cO = cos(O); sO = sin(O); co = cos(o); so = sin(o); ci = cos(i); si = sin(i);
PQW2IJK(1,1,:) = cO.*co-sO.*so.*ci; PQW2IJK(1,2,:) = -cO.*so-sO.*co.*ci; PQW2IJK(1,3,:) = sO.*si;
PQW2IJK(2,1,:) = sO.*co+cO.*so.*ci; PQW2IJK(2,2,:) = -sO.*so+cO.*co.*ci; PQW2IJK(2,3,:) = -cO.*si;
PQW2IJK(3,1,:) = so.*si;            PQW2IJK(3,2,:) = co.*si;             PQW2IJK(3,3,:) = ci;
%Transform rPQW and vPQW to rECI and vECI
r = multiDimMatrixMultiply(PQW2IJK,rPQW)';  
v = multiDimMatrixMultiply(PQW2IJK,vPQW)';
end
function c = multiDimMatrixMultiply(a,b)
c = NaN(size(b));
c(:,1) = sum(bsxfun(@times,a(1,:,:),permute(b,[3 2 1])),2);
c(:,2) = sum(bsxfun(@times,a(2,:,:),permute(b,[3 2 1])),2);
c(:,3) = sum(bsxfun(@times,a(3,:,:),permute(b,[3 2 1])),2);
end

== matlab function IonSatSimulationD/Kalman Filter/IGRF Computation block1/ECI To LLA ==
  data: X_ECEF input; h output; lat output; long output
function [h, lat, long] = fcn(X_ECEF)
    h = 0;
    lat = 0;
    long = 0;
[lat, long, h] = ecef2geod(X_ECEF(1),X_ECEF(2),X_ECEF(3));

== matlab function IonSatSimulationD/Disturbance Torques/Aerodynamic Model/Get Density/ECI To LLA ==
  data: X_ECEF input; h output; lat output; long output
function [h, lat, long] = fcn(X_ECEF)
    h = 0;
    lat = 0;
    long = 0;
[lat, long, h] = ecef2geod(X_ECEF(1),X_ECEF(2),X_ECEF(3));

== matlab function IonSatSimulationD/IGRF Computation block/ECI To LLA ==
  data: X_ECEF input; h output; lat output; long output
function [h, lat, long] = fcn(X_ECEF)
    h = 0;
    lat = 0;
    long = 0;
[lat, long, h] = ecef2geod(X_ECEF(1),X_ECEF(2),X_ECEF(3));

== matlab function IonSatSimulationD/Disturbance Torques/Aerodynamic Model/Get Density/MATLAB Function2 ==
  data: u input; y output
function y = fcn(u)
y = u(6);

== matlab function IonSatSimulationD/Time propagator/UTC to JD ==
  data: Time_UTC input; JD output
function JD = fcn(Time_UTC)

% JD = juliandate(Time_UTC);
JD = Dt2jD(Time_UTC);

== matlab function IonSatSimulationD/Time propagator/JD to UTC ==
  data: JD input; Time_UTC output
function Time_UTC = fcn(JD)
    coder.extrinsic('datetime','datevec');
    Time_UTC = [0,0,0,0,0,0];
Time_UTC =  datevec(datetime(JD,'convertfrom','juliandate'));

== matlab function IonSatSimulationD/Thruster activation/MATLAB Function ==
  data: u input; y output
function y = fcn(u)
time=u(1);
duration=u(2);
initial=u(3);
wait=u(4);
boolean=0;
booleant=0;

if (initial<time)&&(time<(initial+duration))
    boolean=1;
end

if (initial+duration+wait<time)&&(time<(initial+2*duration+wait))
    boolean=1;
end

if (initial+2*(duration+wait)<time)&&(time<(initial+2*(duration+wait)+duration))
    boolean=1;
end

if (initial+3*(duration+wait)<time)&&(time<(initial+3*(duration+wait)+duration))
    boolean=1;
end

y = booleant~=boolean;
